simulink model "L2_Step2"  (R2023a)
settings: Solver=FixedStepDiscrete  StartTime=0.0  StopTime=inf  FixedStep=0.01  RelTol=1e-3
model workspace (MATLAB code in the model file):
  | IgnitionOff = 0;
  | IgnitionACC = 1;
  | IgnitionOnEngineOn = 2;
  | 
  | Active = 1;
  | Not_Active = 0;
  | 
  | 
  | Present = 1;
  | Absent = 0;
settings Model: Creator=Ekrem Fidan  LastModifiedBy=okanduzyel
settings DebuggingCC: UnconnectedInputMsg=warning  UnconnectedOutputMsg=warning  UnconnectedLineMsg=warning
settings ModelReferenceCC: EnableRefExpFcnMdlSchedulingChecks=on
settings RTWCC: DLArmComputeVersion=19.05

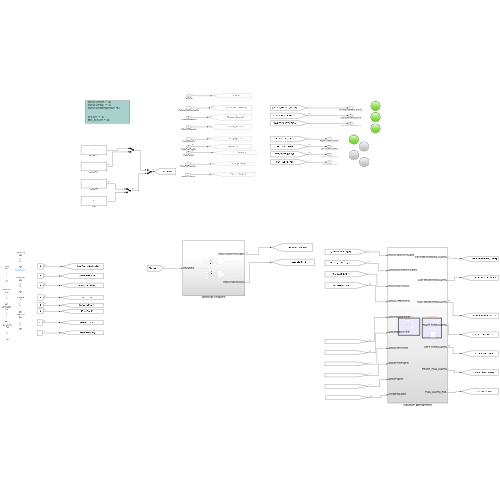
[thumbnail: Simulink's stored preview of the top-level diagram]
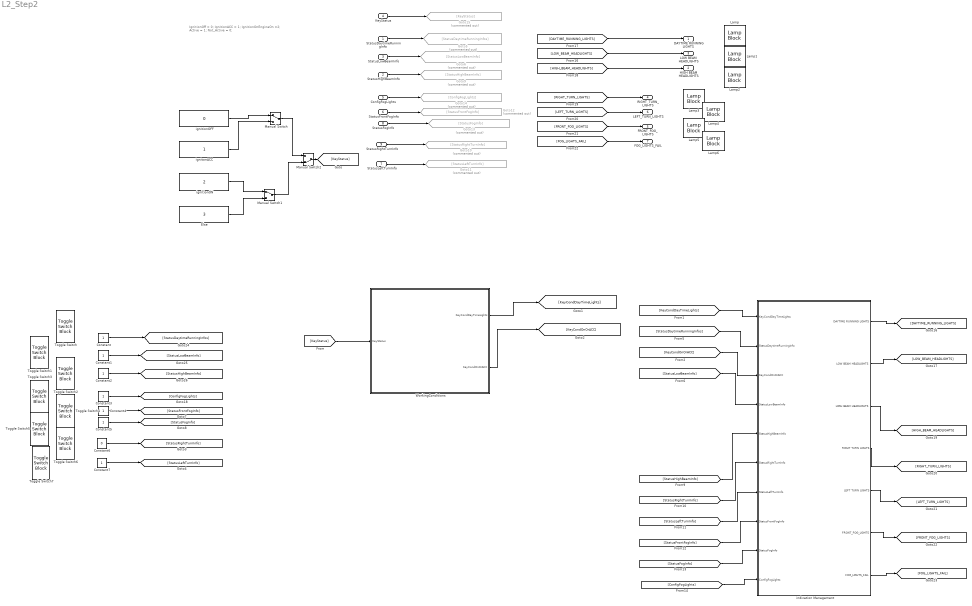
== system L2_Step2 ==
  note: IgnitionOff = 0;
      | IgnitionACC = 1;
      | IgnitionOnEngineOn =2;
      |
      | Active = 1;
      | Not_Active = 0;
  StatusDaytimeRunningInfo : Inport
  StatusHighBeamInfo : Inport  Port=2
  StatusLowBeamInfo : Inport  Port=3
  KeyStatus : Inport  Port=4
  ConfigFogLights : Inport  Port=5
  StatusFrontFogInfo : Inport  Port=6
  StatusLeftTurnInfo : Inport  Port=7
  StatusFogInfo : Inport  Port=8
  StatusRightTurnInfo : Inport  Port=9
  Constant{,1..5,7} (7 alike) : Constant
  Constant6 : Constant  Value=0
  Else : Constant  Value=3  SampleTime=-1
  Goto10 : Goto  Commented=on  GotoTag=StatusRightTurnInfo
  Goto11 : Goto  Commented=on  GotoTag=StatusLeftTurnInfo
  Goto12 : Goto  Commented=on  GotoTag=StatusFrontFogInfo
  Goto13 : Goto  Commented=on  GotoTag=StatusFogInfo
  Goto14 : Goto  Commented=on  GotoTag=ConfigFogLights
  Goto15 : Goto  Commented=on  GotoTag=KeyStatus
  Goto5 : Goto  Commented=on  GotoTag=StatusDaytimeRunningInfos
  Goto6 : Goto  Commented=on  GotoTag=StatusLowBeamInfo
  Goto9 : Goto  Commented=on  GotoTag=StatusHighBeamInfo
  Lamp{,1..6} (7 alike) : LampBlock  LabelPosition=Hide
  Manual Switch : ManualSwitch
  Manual Switch1 : ManualSwitch
  Manual Switch2 : ManualSwitch  CurrentSetting=0
  Toggle Switch{,1..7} (8 alike) : ToggleSwitchBlock
      settings: Values={{'Off', 'On'}, [0 1]}
  WorkingConditions : Subsystem
  ignitionOFF : Constant  Value=0  SampleTime=-1
  ignitionON : Constant  Value=2  SampleTime=-1
  ignitonACC : Constant  SampleTime=-1
  indication Management : Subsystem
  DAYTIME RUNNING LIGHTS : Outport
  HIGH BEAM HEADLIGHTS : Outport  Port=2
  LOW BEAM HEADLIGHTS : Outport  Port=3
  RIGHT_TURN_LIGHTS : Outport  Port=4
  FRONT_FOG_LIGHTS : Outport  Port=5
  LEFT_TURN_LIGHTS : Outport  Port=6
  FOG_LIGHTS_FAIL : Outport  Port=7
  wires:
  ignitionOFF/1 -> Manual Switch/1
  ignitonACC/1 -> Manual Switch/2
  ignitionON/1 -> Manual Switch1/1
  Else/1 -> Manual Switch1/2
  Manual Switch/1 -> Manual Switch2/1
  Manual Switch1/1 -> Manual Switch2/2
  Manual Switch2/1 -> [KeyStatus]
  [KeyStatus] -> WorkingConditions/1(KeyStatus)
  WorkingConditions/1(KeyCondDayTimeLights) -> [KeyCondDayTimeLights]
  [KeyCondDayTimeLights] -> indication Management/1(KeyCondDayTimeLights)
  WorkingConditions/2(KeyCondOnOrACC) -> [KeyCondOnOrACC]
  [KeyCondOnOrACC] -> indication Management/3(KeyCondOnOrACC)
  [StatusDaytimeRunningInfos] -> indication Management/2(StatusDaytimeRunningInfo)
  [StatusLowBeamInfo] -> indication Management/4(StatusLowBeamInfo)
  [StatusHighBeamInfo] -> indication Management/5(StatusHighBeamInfo)
  [StatusRightTurnInfo] -> indication Management/6(StatusRightTurnInfo)
  [StatusLeftTurnInfo] -> indication Management/7(StatusLeftTurnInfo)
  [StatusFrontFogInfo] -> indication Management/8(StatusFrontFogInfo)
  [StatusFogInfo] -> indication Management/9(StatusFogInfo)
  [ConfigFogLights] -> indication Management/10(ConfigFogLights)
  StatusDaytimeRunningInfo/1 -> Goto5/1
  StatusLowBeamInfo/1 -> Goto6/1
  StatusHighBeamInfo/1 -> Goto9/1
  KeyStatus/1 -> Goto15/1
  ConfigFogLights/1 -> Goto14/1
  StatusFogInfo/1 -> Goto13/1
  StatusFrontFogInfo/1 -> Goto12/1
  StatusLeftTurnInfo/1 -> Goto11/1
  StatusRightTurnInfo/1 -> Goto10/1
  indication Management/1(DAYTIME RUNNING LIGHTS) -> [DAYTIME_RUNNING_LIGHTS]
  indication Management/2(LOW BEAM HEADLIGHTS) -> [LOW_BEAM_HEADLIGHTS]
  indication Management/3(HIGH BEAM HEADLIGHTS) -> [HIGH_BEAM_HEADLIGHTS]
  indication Management/4(RIGHT TURN LIGHTS) -> [RIGHT_TURN_LIGHTS]
  indication Management/5(LEFT TURN LIGHTS) -> [LEFT_TURN_LIGHTS]
  indication Management/6(FRONT_FOG_LIGHTS) -> [FRONT_FOG_LIGHTS]
  indication Management/7(FOG_LIGHTS_FAIL) -> [FOG_LIGHTS_FAIL]
  [DAYTIME_RUNNING_LIGHTS] -> DAYTIME RUNNING LIGHTS/1
  [LOW_BEAM_HEADLIGHTS] -> LOW BEAM HEADLIGHTS/1
  [HIGH_BEAM_HEADLIGHTS] -> HIGH BEAM HEADLIGHTS/1
  [LEFT_TURN_LIGHTS] -> LEFT_TURN_LIGHTS/1
  [RIGHT_TURN_LIGHTS] -> RIGHT_TURN_LIGHTS/1
  [FRONT_FOG_LIGHTS] -> FRONT_FOG_LIGHTS/1
  [FOG_LIGHTS_FAIL] -> FOG_LIGHTS_FAIL/1
  Constant5/1 -> [StatusFogInfo]
  Constant1/1 -> [StatusLowBeamInfo]
  Constant7/1 -> [StatusLeftTurnInfo]
  Constant6/1 -> [StatusRightTurnInfo]
  Constant/1 -> [StatusDaytimeRunningInfos]
  Constant2/1 -> [StatusHighBeamInfo]
  Constant3/1 -> [ConfigFogLights]
  Constant4/1 -> [StatusFrontFogInfo]

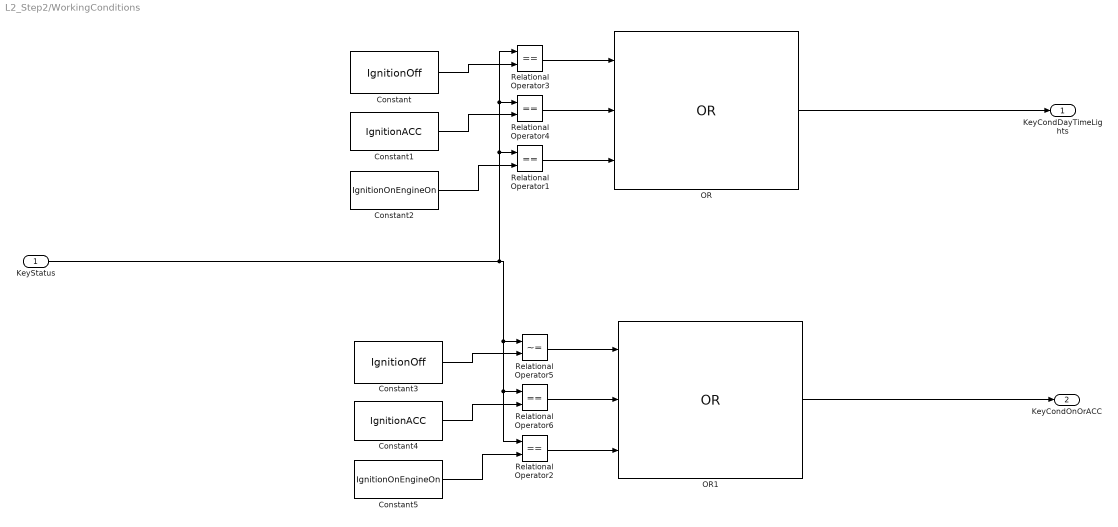
== system L2_Step2/WorkingConditions ==
  KeyStatus : Inport
  Constant : Constant  Value=IgnitionOff  SampleTime=-1
  Constant1 : Constant  Value=IgnitionACC  SampleTime=-1
  Constant2 : Constant  Value=IgnitionOnEngineOn  SampleTime=-1
  Constant3 : Constant  Value=IgnitionOff  SampleTime=-1
  Constant4 : Constant  Value=IgnitionACC  SampleTime=-1
  Constant5 : Constant  Value=IgnitionOnEngineOn  SampleTime=-1
  OR : Logic  Operator=OR  Inputs=3  IconShape=distinctive  AllPortsSameDT=off  OutDataTypeStr=boolean
  OR1 : Logic  Operator=OR  Inputs=3  IconShape=distinctive  AllPortsSameDT=off  OutDataTypeStr=boolean
  Relational Operator{1..4,6} (5 alike) : RelationalOperator  Operator===  OutDataTypeStr=boolean  RndMeth=Simplest  InputSameDT=off
  Relational Operator5 : RelationalOperator  Operator=~=  OutDataTypeStr=boolean  RndMeth=Simplest  InputSameDT=off
  KeyCondDayTimeLights : Outport
  KeyCondOnOrACC : Outport  Port=2
  wires:
  Constant1/1 -> Relational Operator4/2
  Relational Operator3/1 -> OR/1
  Constant/1 -> Relational Operator3/2
  Relational Operator4/1 -> OR/2
  OR/1 -> KeyCondDayTimeLights/1
  Relational Operator1/1 -> OR/3
  Constant2/1 -> Relational Operator1/2
  Constant5/1 -> Relational Operator2/2
  Relational Operator2/1 -> OR1/3
  OR1/1 -> KeyCondOnOrACC/1
  Relational Operator6/1 -> OR1/2
  Constant3/1 -> Relational Operator5/2
  Relational Operator5/1 -> OR1/1
  Constant4/1 -> Relational Operator6/2
  KeyStatus/1 -> Relational Operator2/1, Relational Operator6/1, Relational Operator5/1, Relational Operator1/1, Relational Operator4/1, Relational Operator3/1

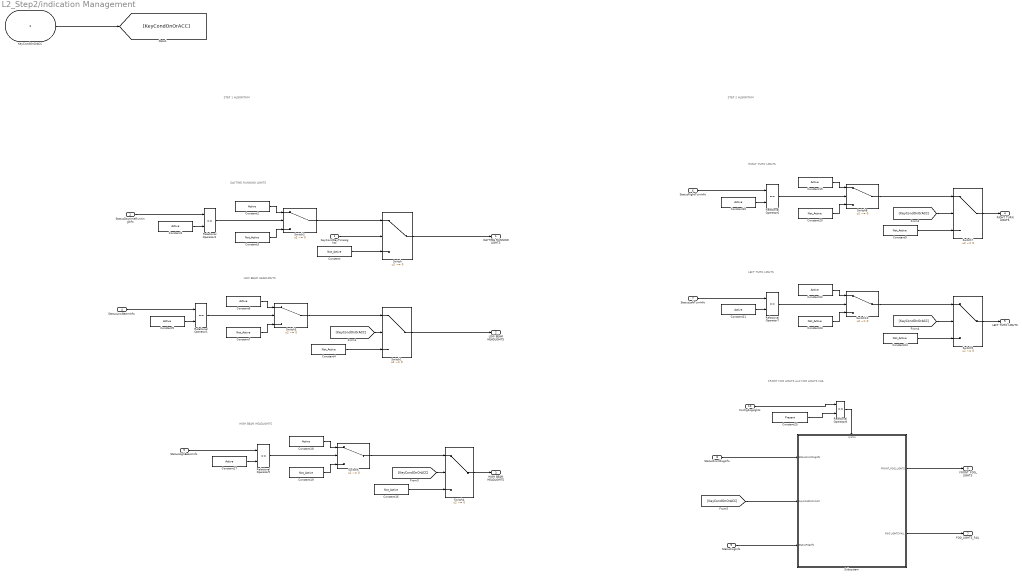
== system L2_Step2/indication Management ==
  note: STEP 1 ALGORITHM
  note: DAYTIME RUNNING LIGHTS
  note: LOW BEAM HEADLIGHTS
  note: HIGH BEAM HEADLIGHTS
  note: RIGHT TURN LIGHTS
  note: LEFT TURN LIGHTS
  note: FRONT FOG LIGHTS and FOG LIGHTS FAIL
  note: STEP 2 ALGORITHM
  KeyCondDayTimeLights : Inport
  StatusDaytimeRunningInfo : Inport  Port=2
  KeyCondOnOrACC : Inport  Port=3
  StatusLowBeamInfo : Inport  Port=4
  StatusHighBeamInfo : Inport  Port=5
  StatusRightTurnInfo : Inport  Port=6
  StatusLeftTurnInfo : Inport  Port=7
  StatusFrontFogInfo : Inport  Port=8
  StatusFogInfo : Inport  Port=9
  ConfigFogLights : Inport  Port=10
  Constant{,3..4,7,9,16,19..20,23..24} (10 alike) : Constant  Value=Not_Active  SampleTime=-1
  Constant{1..2,5..6,10,15,17..18,21..22} (10 alike) : Constant  Value=Active  SampleTime=-1
  Constant25 : Constant  Value=Present  SampleTime=-1
  Relational Operator{1,3,5..8} (6 alike) : RelationalOperator  Operator===  OutDataTypeStr=boolean  RndMeth=Simplest  InputSameDT=off
  Subsystem : Subsystem
  Switch{,1..4,6..10} (10 alike) : Switch  Criteria=u2 ~= 0  SaturateOnIntegerOverflow=off  InputSameDT=off
  DAYTIME RUNNING LIGHTS : Outport
  LOW BEAM HEADLIGHTS : Outport  Port=2
  HIGH BEAM HEADLIGHTS : Outport  Port=3
  RIGHT TURN LIGHTS : Outport  Port=4
  LEFT TURN LIGHTS : Outport  Port=5
  FRONT_FOG_LIGHTS : Outport  Port=6
  FOG_LIGHTS_FAIL : Outport  Port=7
  wires:
  Constant1/1 -> Relational Operator3/2
  KeyCondDayTimeLights/1 -> Switch/2
  Switch2/1 -> Switch/1
  Constant2/1 -> Switch2/1
  Switch/1 -> DAYTIME RUNNING LIGHTS/1
  Constant/1 -> Switch/3
  Constant3/1 -> Switch2/3
  Relational Operator3/1 -> Switch2/2
  StatusDaytimeRunningInfo/1 -> Relational Operator3/1
  StatusLowBeamInfo/1 -> Relational Operator1/1
  Relational Operator1/1 -> Switch3/2
  Constant7/1 -> Switch3/3
  Constant4/1 -> Switch1/3
  Constant6/1 -> Switch3/1
  Switch3/1 -> Switch1/1
  [KeyCondOnOrACC] -> Switch1/2
  Constant5/1 -> Relational Operator1/2
  Switch1/1 -> LOW BEAM HEADLIGHTS/1
  KeyCondOnOrACC/1 -> [KeyCondOnOrACC]
  Constant17/1 -> Relational Operator5/2
  [KeyCondOnOrACC] -> Switch4/2
  Switch6/1 -> Switch4/1
  Constant18/1 -> Switch6/1
  Constant16/1 -> Switch4/3
  Constant19/1 -> Switch6/3
  Relational Operator5/1 -> Switch6/2
  StatusHighBeamInfo/1 -> Relational Operator5/1
  Switch4/1 -> HIGH BEAM HEADLIGHTS/1
  Switch7/1 -> RIGHT TURN LIGHTS/1
  Constant9/1 -> Switch7/3
  StatusRightTurnInfo/1 -> Relational Operator6/1
  Constant20/1 -> Switch8/3
  Relational Operator6/1 -> Switch8/2
  Constant10/1 -> Relational Operator6/2
  Switch8/1 -> Switch7/1
  Constant15/1 -> Switch8/1
  [KeyCondOnOrACC] -> Switch7/2
  [KeyCondOnOrACC] -> Switch9/2
  Constant22/1 -> Switch10/1
  Switch10/1 -> Switch9/1
  Constant21/1 -> Relational Operator7/2
  Relational Operator7/1 -> Switch10/2
  Constant23/1 -> Switch10/3
  StatusLeftTurnInfo/1 -> Relational Operator7/1
  Constant24/1 -> Switch9/3
  Switch9/1 -> LEFT TURN LIGHTS/1
  StatusFrontFogInfo/1 -> Subsystem/1(StatusFrontFogInfo)
  [KeyCondOnOrACC] -> Subsystem/2(KeyCondOnOrACC)
  StatusFogInfo/1 -> Subsystem/3(StatusFogInfo)
  Subsystem/1(FRONT_FOG_LIGHTS) -> FRONT_FOG_LIGHTS/1
  Subsystem/2(FOG LIGHTS FAIL) -> FOG_LIGHTS_FAIL/1
  ConfigFogLights/1 -> Relational Operator8/1
  Constant25/1 -> Relational Operator8/2
  Relational Operator8/1 -> Subsystem/Enable

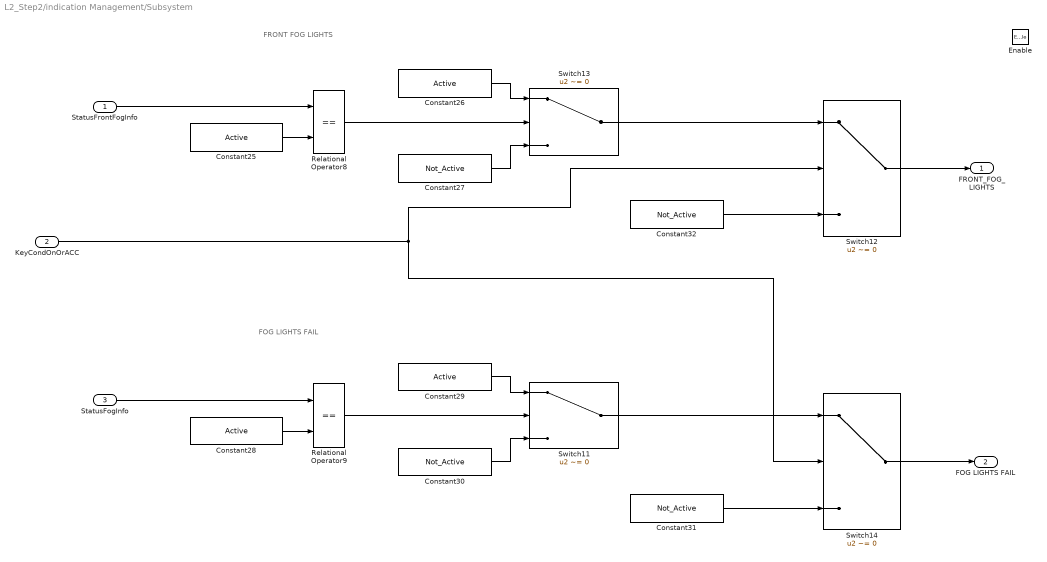
== system L2_Step2/indication Management/Subsystem ==
  note: FOG LIGHTS FAIL
  note: FRONT FOG LIGHTS
  StatusFrontFogInfo : Inport
  KeyCondOnOrACC : Inport  Port=2
  StatusFogInfo : Inport  Port=3
  Enable : EnablePort
  Constant{25..26,28..29} (4 alike) : Constant  Value=Active  SampleTime=-1
  Constant{27,30..32} (4 alike) : Constant  Value=Not_Active  SampleTime=-1
  Relational Operator8 : RelationalOperator  Operator===  OutDataTypeStr=boolean  RndMeth=Simplest  InputSameDT=off
  Relational Operator9 : RelationalOperator  Operator===  OutDataTypeStr=boolean  RndMeth=Simplest  InputSameDT=off
  Switch{11..14} (4 alike) : Switch  Criteria=u2 ~= 0  SaturateOnIntegerOverflow=off  InputSameDT=off
  FRONT_FOG_LIGHTS : Outport
  FOG LIGHTS FAIL : Outport  Port=2
  wires:
  Constant28/1 -> Relational Operator9/2
  Constant25/1 -> Relational Operator8/2
  Constant30/1 -> Switch11/3
  Constant31/1 -> Switch14/3
  StatusFrontFogInfo/1 -> Relational Operator8/1
  Constant32/1 -> Switch12/3
  Switch11/1 -> Switch14/1
  Switch12/1 -> FRONT_FOG_LIGHTS/1
  Constant29/1 -> Switch11/1
  KeyCondOnOrACC/1 -> Switch12/2, Switch14/2
  Constant26/1 -> Switch13/1
  Switch13/1 -> Switch12/1
  Constant27/1 -> Switch13/3
  Relational Operator8/1 -> Switch13/2
  Switch14/1 -> FOG LIGHTS FAIL/1
  Relational Operator9/1 -> Switch11/2
  StatusFogInfo/1 -> Relational Operator9/1
